simulink model "RL_DB_Scenarios"  (R2018a)
settings: Solver=FixedStepAuto  StartTime=0.0  StopTime=Tfinal  MaxStep=Ts  RelTol=1e-3
values from neighbouring files (symbols this model uses):
  Fline = 50    [Param.m]
  Fs = 20000    [Param.m]
  FStepTime = 0.105    [Param.m]
  Lload = Xload / 2 / pi / Fline    (= 318309.886184)    [Param.m]
  Rdiodebridge = 0.5 * Vline^2 / Pdiodebridge    (= 1)    [Param.m]
  Rload = Vline^2 / Pload    (= 100000000)    [Param.m]
  SineDistActive = 1    [Param.m]
  SineDistActTime = 0.105    [Param.m]
  SineDistAmp = 0.5    [Param.m]
  SineDistFreq = sinefrequency    (= 0.666666666667)    [Param.m]
  SineDistPhase = -SineDistActTime * 2 * pi * SineDistFreq    (= -0.439822971503)    [Param.m]
  StepActive = 1    [Param.m]
  StepAmp = -(SampPerPeriod+4)/SampPerPeriod*Fline+Fline    (= -0.5)    [Param.m]
  Ts = 1 / Fs    (= 5e-05)    [Param.m]
  Vamp = Vline * 2^0.5    (= 1.41421356237)    [Param.m]
undefined symbols (not defined in the file or in its folder): LconvtrafoH
libraries: powerlib x12, CPTLibrary x4
settings Model: Creator=daniemot  LastModifiedBy=daniemot

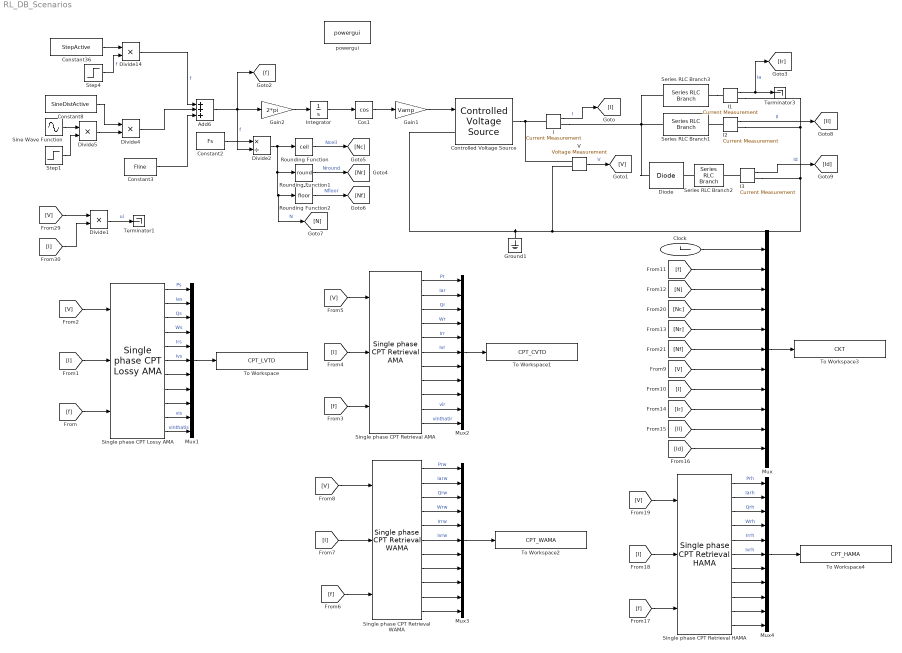
== system RL_DB_Scenarios ==
  Add6 : Sum  Inputs=+++
  Clock : Clock
  Constant2 : Constant  Value=Fs
  Constant3 : Constant  Value=Fline
  Constant36 : Constant  Value=StepActive
  Constant8 : Constant  Value=SineDistActive
  Controlled Voltage Source : powerlib/Electrical Sources/Controlled Voltage Source  Initialize=on  Source_Type=DC  Amplitude=0  Phase=0  Frequency=0  Measurements=None
  Cos1 : Trigonometry  Operator=cos
  Diode : powerlib/Power Electronics/Diode  Ron=0.001  Lon=0  Vf=0.00000001  IC=0  UseSnubber=0  Rs=500  Cs=0  Measurements=off
  Divide{1,4..5,14} (4 alike) : Product  Inputs=**
  Divide2 : Product  Inputs=*/
  Gain1 : Gain  Gain=Vamp
  Gain2 : Gain  Gain=2*pi
  Ground1 : powerlib/Elements/Ground  LConnTagsString=a
      settings: SourceProductName=Simscape Electrical
  I{,1..3} (4 alike) : powerlib/Measurements/Current Measurement  PhasorSimulation=off  OutputType=Complex  PSBequivalent=0
  Integrator : Integrator
  Mux{,1..4} (5 alike) : Mux  Inputs=11
  Rounding Function : Rounding  Operator=ceil
  Rounding Function1 : Rounding  Operator=round
  Rounding Function2 : Rounding
  Series RLC Branch1 : powerlib/Elements/Series RLC Branch  LConnTagsString=__new0  RConnTagsString=__new0  BranchType=L  Resistance=1  Inductance=Lload  SetiL0=on  InitialCurrent=0  Capacitance=0  Setx0=off  InitialVoltage=0  Measurements=None
  Series RLC Branch2 : powerlib/Elements/Series RLC Branch  LConnTagsString=__new0  RConnTagsString=__new0  BranchType=R  Resistance=Rdiodebridge  Inductance=LconvtrafoH  SetiL0=off  InitialCurrent=Iloadbridgeinitial  Capacitance=0  Setx0=off  InitialVoltage=0  Measurements=None
  Series RLC Branch3 : powerlib/Elements/Series RLC Branch  LConnTagsString=__new0  RConnTagsString=__new0  BranchType=R  Resistance=Rload  Inductance=LconvtrafoH  SetiL0=off  InitialCurrent=Iloadbridgeinitial  Capacitance=0  Setx0=off  InitialVoltage=0  Measurements=None
  Sine Wave Function : Sin  Amplitude=SineDistAmp  Frequency=SineDistFreq*2*pi  Phase=SineDistPhase  SampleTime=0
  Single phase CPT Lossy AMA : CPTLibrary/CPT Single Phase/Single phase CPT Lossy AMA  NbSize=MaxSampPerPeriod  Ts=Ts
  Single phase CPT Retrieval AMA : CPTLibrary/CPT Single Phase/Single phase CPT Retrieval AMA  NbSize=MaxSampPerPeriod  Ts=Ts
  Single phase CPT Retrieval HAMA : CPTLibrary/CPT Single Phase/Single phase CPT Retrieval HAMA  NbSize=MaxSampPerPeriod  Ts=Ts
  Single phase CPT Retrieval WAMA : CPTLibrary/CPT Single Phase/Single phase CPT Retrieval WAMA  NbSize=MaxSampPerPeriod  Ts=Ts
  Step1 : Step  Time=SineDistActTime  SampleTime=Ts
  Step4 : Step  Time=FStepTime  After=StepAmp  SampleTime=Ts
  Terminator1 : Terminator
  Terminator3 : Terminator
  To Workspace : ToWorkspace  VariableName=CPT_LVTD  SampleTime=Ts
  To Workspace1 : ToWorkspace  VariableName=CPT_CVTD  SampleTime=Ts
  To Workspace2 : ToWorkspace  VariableName=CPT_WAMA  SampleTime=Ts
  To Workspace3 : ToWorkspace  VariableName=CKT  SampleTime=Ts
  To Workspace4 : ToWorkspace  VariableName=CPT_HAMA  SampleTime=Ts
  V : powerlib/Measurements/Voltage Measurement  PhasorSimulation=off  OutputType=Complex  PSBequivalent=0
  powergui : powerlib/powergui  Priority=1  SimulationMode=Discrete  SampleTime=Ts/100  frequency=60  Iterations=50  frequencyindice=0  Pbase=100e6  ErrMax=1e-4  UnitsV=kV  UnitsW=MW  buscounter=0  FunctionMessages=off  echomessages=off  EnableUseOfTLC=off  CurrentSourceSwitches=off  DisableSnubberDevices=off  DisableRonSwitches=off  DisableVfSwitches=off  DisplayEquations=off  SolverType=Tustin/Backward Euler (TBE)  Interpol=off  ExternalGateDelay=off  methode=off  Ts=100  x0status=zero  SPID=off  SwTol=0  HookPort=off  RestoreLinks=warning  ResistiveCurrentMeasurement=off  Frange=[0:2:500]  Ylog=off  Xlog=on  ShowGrid=off  save=off  variable=ZData  structure=0  ZoomFFT=off  StartTime=0.0  cycles=1  DisplayStyle=1  fundamental=60  FreqAxis=off  MaxFrequency=1000  frequencyindicesteady=1  RmsSteady=1  display=off
  wires:
  Divide14/1 -> Add6/1  "f"
  Step4/1 -> Divide14/2  "f"
  Constant36/1 -> Divide14/1
  Add6/1 -> [f], Divide2/2, Gain2/1  "f"
  Divide2/1 -> [N], Rounding Function2/1, Rounding Function1/1, Rounding Function/1  "N"
  Gain2/1 -> Integrator/1
  I/1 -> [I]  "I"
  V/1 -> [V]  "V"
  I1/1 -> [Ir], Terminator3/1  "Ia"
  I2/1 -> [Il]  "Il"
  Integrator/1 -> Cos1/1
  Cos1/1 -> Gain1/1
  Gain1/1 -> Controlled Voltage Source/1
  Constant8/1 -> Divide4/1
  Divide4/1 -> Add6/2
  Sine Wave Function/1 -> Divide5/1
  Step1/1 -> Divide5/2
  Divide5/1 -> Divide4/2
  Constant3/1 -> Add6/3
  Constant2/1 -> Divide2/1
  Rounding Function/1 -> [Nc]  "Nceil"
  I3/1 -> [Id]  "Id"
  [f] -> Single phase CPT Lossy AMA/3
  [I] -> Single phase CPT Lossy AMA/2
  [V] -> Single phase CPT Lossy AMA/1
  Single phase CPT Retrieval AMA/1 -> Mux2/1  "Pr"
  Single phase CPT Retrieval AMA/4 -> Mux2/4  "Wr"
  Single phase CPT Retrieval AMA/3 -> Mux2/3  "Qr"
  Single phase CPT Retrieval AMA/6 -> Mux2/6  "Ivr"
  Single phase CPT Retrieval AMA/5 -> Mux2/5  "Irr"
  Single phase CPT Retrieval AMA/2 -> Mux2/2  "Iar"
  Single phase CPT Retrieval WAMA/1 -> Mux3/1  "Prw"
  Single phase CPT Retrieval WAMA/4 -> Mux3/4  "Wrw"
  Single phase CPT Retrieval WAMA/3 -> Mux3/3  "Qrw"
  Single phase CPT Retrieval WAMA/6 -> Mux3/6  "Ivrw"
  Single phase CPT Retrieval WAMA/5 -> Mux3/5  "Irrw"
  Single phase CPT Retrieval WAMA/2 -> Mux3/2  "Iarw"
  [f] -> Single phase CPT Retrieval AMA/3
  [V] -> Single phase CPT Retrieval AMA/1
  [I] -> Single phase CPT Retrieval AMA/2
  [f] -> Single phase CPT Retrieval WAMA/3
  [V] -> Single phase CPT Retrieval WAMA/1
  [I] -> Single phase CPT Retrieval WAMA/2
  Rounding Function1/1 -> [Nr]  "Nround"
  Rounding Function2/1 -> [Nf]  "Nfloor"
  Mux/1 -> To Workspace3/1
  [f] -> Mux/2
  [N] -> Mux/3
  [Nr] -> Mux/5
  [V] -> Mux/7
  [I] -> Mux/8
  [Ir] -> Mux/9
  [Il] -> Mux/10
  [Id] -> Mux/11
  Mux1/1 -> To Workspace/1
  [V] -> Divide1/1
  [I] -> Divide1/2
  Divide1/1 -> Terminator1/1  "ui"
  Single phase CPT Retrieval AMA/10 -> Mux2/10  "vir"
  Single phase CPT Retrieval AMA/11 -> Mux2/11  "vinthatir"
  Single phase CPT Lossy AMA/1 -> Mux1/1  "Ps"
  Single phase CPT Lossy AMA/2 -> Mux1/2  "Ias"
  Single phase CPT Lossy AMA/3 -> Mux1/3  "Qs"
  Single phase CPT Lossy AMA/4 -> Mux1/4  "Ws"
  Single phase CPT Lossy AMA/5 -> Mux1/5  "Irs"
  Single phase CPT Lossy AMA/6 -> Mux1/6  "Ivs"
  Single phase CPT Lossy AMA/7 -> Mux1/7
  Single phase CPT Lossy AMA/8 -> Mux1/8
  Single phase CPT Lossy AMA/9 -> Mux1/9
  Single phase CPT Lossy AMA/10 -> Mux1/10  "vis"
  Single phase CPT Lossy AMA/11 -> Mux1/11  "vinthatis"
  Mux2/1 -> To Workspace1/1
  Single phase CPT Retrieval AMA/7 -> Mux2/7
  Single phase CPT Retrieval AMA/8 -> Mux2/8
  Single phase CPT Retrieval AMA/9 -> Mux2/9
  Mux3/1 -> To Workspace2/1
  Single phase CPT Retrieval WAMA/7 -> Mux3/7
  Single phase CPT Retrieval WAMA/8 -> Mux3/8
  Single phase CPT Retrieval WAMA/9 -> Mux3/9
  Single phase CPT Retrieval WAMA/10 -> Mux3/10
  Single phase CPT Retrieval WAMA/11 -> Mux3/11
  [V] -> Single phase CPT Retrieval HAMA/1
  [I] -> Single phase CPT Retrieval HAMA/2
  [f] -> Single phase CPT Retrieval HAMA/3
  Single phase CPT Retrieval HAMA/10 -> Mux4/10
  Single phase CPT Retrieval HAMA/11 -> Mux4/11
  Mux4/1 -> To Workspace4/1
  Single phase CPT Retrieval HAMA/5 -> Mux4/5  "Irrh"
  Single phase CPT Retrieval HAMA/9 -> Mux4/9
  Single phase CPT Retrieval HAMA/7 -> Mux4/7
  Single phase CPT Retrieval HAMA/6 -> Mux4/6  "Ivrh"
  Single phase CPT Retrieval HAMA/4 -> Mux4/4  "Wrh"
  Single phase CPT Retrieval HAMA/2 -> Mux4/2  "Iarh"
  Single phase CPT Retrieval HAMA/8 -> Mux4/8
  Single phase CPT Retrieval HAMA/1 -> Mux4/1  "Prh"
  Single phase CPT Retrieval HAMA/3 -> Mux4/3  "Qrh"
  Clock/1 -> Mux/1
  [Nc] -> Mux/4
  [Nf] -> Mux/6
  connections:
  I2/RConn1 -- I3/RConn1 -- V/LConn2 -- Ground1/LConn1 -- Controlled Voltage Source/LConn1 -- I1/RConn1
  Controlled Voltage Source/RConn1 -- V/LConn1 -- I/LConn1
  I/RConn1 -- Diode/LConn1 -- Series RLC Branch1/LConn1 -- Series RLC Branch3/LConn1
  I2/LConn1 -- Series RLC Branch1/RConn1
  Series RLC Branch3/RConn1 -- I1/LConn1
  Series RLC Branch2/LConn1 -- Diode/RConn1
  I3/LConn1 -- Series RLC Branch2/RConn1
